simulink model "Case2WithTime"  (R2023b)
settings: Solver=VariableStepAuto  StartTime=0.0  StopTime=10.0  RelTol=1e-3
settings Model: Creator=iceki  LastModifiedBy=iceki

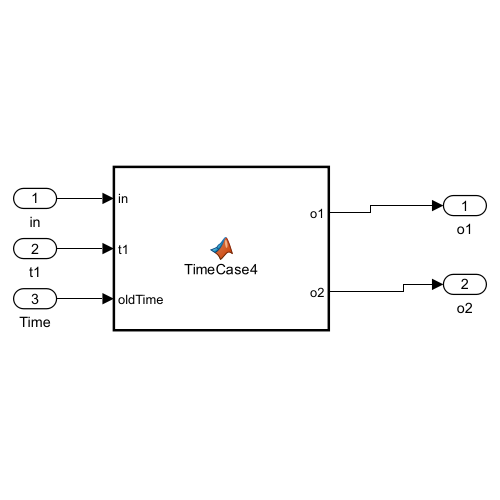
[thumbnail: Simulink's stored preview of the top-level diagram]
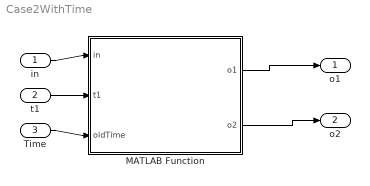
== system Case2WithTime ==
  in : Inport
  t1 : Inport  Port=2
  Time : Inport  Port=3
  MATLAB Function : MATLAB Function  TreatAsAtomicUnit=on
  o1 : Outport
  o2 : Outport  Port=2
  wires:
  in/1 -> MATLAB Function/1(in)
  t1/1 -> MATLAB Function/2(t1)
  MATLAB Function/1(o1) -> o1/1
  MATLAB Function/2(o2) -> o2/1
  Time/1 -> MATLAB Function/3(oldTime)

== matlab function Case2WithTime/MATLAB Function ==
  data: in input; o1 output; t1 input; o2 output; oldTime input
function [o1,o2] = TimeCase4(in,t1,oldTime)


o1 = -1;
o2 = -1;

%rng('shuffle');
x = rand*100;

if 0  <= x && x < t1
    o1 = in + oldTime;
else
    o2 = in + oldTime;
end

if in == -1
    o1 = -1
    o2 = -1
end
